simulink model "soc_WLAN_fpga"  (R2024b)
settings: Solver=FixedStepDiscrete  StartTime=0.0  StopTime=stopTime  RelTol=1e-3
PreLoadFcn:
  | addpath(fullfile(matlabroot,'toolbox','whdl','whdlexamples','whdlexamples'));
InitFcn:
  | addpath(fullfile(matlabroot,'toolbox','whdl','whdlexamples','whdlexamples'));
model workspace (MAT data in the model file):
  socvcb : containers.Map (value not decoded)
undefined symbols (not defined in the file): Add, bitRatePerOfdmSym, chanBW, coe, cpLen, dataUpsampleFactor, DelayValMaxNsdMinusLastPilotSc, DescramblerInitialSeed, designMultirateFIR, fftLen, filterLatency, filterUpsampleFactor, Fs, Hd, HT_MFMCS0, HT_MFMCS1, HT_MFMCS2, HT_MFMCS3, HT_MFMCS4, HT_MFMCS5, HT_MFMCS6, HT_MFMCS7, HTUnUsedScInd, inputSamplingRate, interp_coeff, maxPilotRefCounterVale, maxPilotsRef, maxPilotsRefNonHT, Ncol_HT, Ncol_NonHT, noDataSubCarriers, Non_HTMCS0, Non_HTMCS1, Non_HTMCS2, Non_HTMCS3, Non_HTMCS4, Non_HTMCS5, Non_HTMCS6, Non_HTMCS7, Nrow_HT, Nrow_NonHT, numDSC_HT, numDSC_HT_vhtSigB, numDSC_NonHT, numDscHT, numDscNonHT, numOfBitsPerOFDMSym, numOfDataBitsPerOFDMSym, numPilots, numScHT, numSCS_HT, numSCS_NonHT, pnSeq, QAM, rxDownsampleFactor, secondPIdx_HT, secondPIdx_NonHT, Shift, VHTMCS0, VHTMCS1 ... (+7)
libraries: hdlsllib x267, simulink x210, dspsigops x22, whdlutilities x10, whdlmod x9, dsphdlfiltering2 x5, dsphdlmathfun2 x4, whdledac x3, hwlogicconnlib x2, commhdlcrc x2, dsphdlsigops2 x2
(part 8 of 14)

== system soc_WLAN_fpga/WLAN/WLAN HDL/WLAN_Tx_Rx/WLAN_Rx/WLANHDLReceiver/FrameFormatDetectionAndSignalRecovery/SignalBitRecovery/Deinterleaver Block/Write Logic ==
  start : Inport
  valid : Inport  Port=2
  end : Inport  Port=3
  Generate Write Address : Subsystem
  Handle Input Control Signals : Subsystem
  wrAddr : Outport
  wrValid : Outport  Port=2
  count : Outport  Port=3
  endOut : Outport  Port=4
  endReady : Outport  Port=5
  wires:
  Handle Input Control Signals/4(endReady) -> endReady/1
  end/1 -> Handle Input Control Signals/3(end)
  valid/1 -> Handle Input Control Signals/2(valid)
  Generate Write Address/1(wrAddr) -> wrAddr/1
  Handle Input Control Signals/2(countEnb) -> Generate Write Address/2(enb), wrValid/1
  start/1 -> Handle Input Control Signals/1(start)
  Handle Input Control Signals/3(endOut) -> Generate Write Address/3(end), endOut/1
  Handle Input Control Signals/1(reset) -> Generate Write Address/1(rst)
  Generate Write Address/2(count) -> count/1

== system soc_WLAN_fpga/WLAN/WLAN HDL/WLAN_Tx_Rx/WLAN_Rx/WLANHDLReceiver/HT_VHTCPEEstAndCorrection/CPECorrector/Reciprocal/Function Impl ==
  switch : Inport
  LUTAddr : Inport  Port=2
  Delay{6..8,10,15..16} (6 alike) : Delay
  Delay9 : Delay  DelayLength=1
  LUT1 : LookupNDDirect  NumberOfTableDimensions=1  Table=LUT(:,1)  DiagnosticForOutOfRangeInput=Error
  LUT2 : LookupNDDirect  NumberOfTableDimensions=1  Table=LUT(:,2)  DiagnosticForOutOfRangeInput=Error
  Multiport Switch : MultiPortSwitch  DataPortOrder=Zero-based contiguous  Inputs=2  zeroidx=on  SaturateOnIntegerOverflow=off  InputSameDT=off
  functionValues : Outport
  wires:
  LUTAddr/1 -> Delay7/1, Delay6/1
  Delay15/1 -> Multiport Switch/2
  Delay16/1 -> Multiport Switch/3
  Delay10/1 -> Multiport Switch/1
  Delay9/1 -> functionValues/1
  LUT2/1 -> Delay15/1
  LUT1/1 -> Delay16/1
  switch/1 -> Delay8/1
  Delay8/1 -> Delay10/1
  Delay7/1 -> LUT2/1
  Delay6/1 -> LUT1/1
  Multiport Switch/1 -> Delay9/1

== system soc_WLAN_fpga/WLAN/WLAN HDL/WLAN_Tx_Rx/WLAN_Rx/WLANHDLReceiver/NonHTCPEEstAndCorrection/CPECorrector/Reciprocal/Function Impl ==
  switch : Inport
  LUTAddr : Inport  Port=2
  Delay{6..8,10,15..16} (6 alike) : Delay
  Delay9 : Delay  DelayLength=1
  LUT1 : LookupNDDirect  NumberOfTableDimensions=1  Table=LUT(:,1)  DiagnosticForOutOfRangeInput=Error
  LUT2 : LookupNDDirect  NumberOfTableDimensions=1  Table=LUT(:,2)  DiagnosticForOutOfRangeInput=Error
  Multiport Switch : MultiPortSwitch  DataPortOrder=Zero-based contiguous  Inputs=2  zeroidx=on  SaturateOnIntegerOverflow=off  InputSameDT=off
  functionValues : Outport
  wires:
  LUTAddr/1 -> Delay7/1, Delay6/1
  Delay15/1 -> Multiport Switch/2
  Delay16/1 -> Multiport Switch/3
  Delay10/1 -> Multiport Switch/1
  Delay9/1 -> functionValues/1
  LUT2/1 -> Delay15/1
  LUT1/1 -> Delay16/1
  switch/1 -> Delay8/1
  Delay8/1 -> Delay10/1
  Delay7/1 -> LUT2/1
  Delay6/1 -> LUT1/1
  Multiport Switch/1 -> Delay9/1

== system soc_WLAN_fpga/WLAN/WLAN HDL/WLAN_Tx_Rx/WLAN_Rx/WLANHDLReceiver/WLANTimeAndFrequencySynchronization/Coarse CFO Estimation and Correction/Coarse CFO Estimation/averager ==
  corrIn : Inport
  load : Inport  Port=2
  rst : Inport  Port=3
  Compare To Constant : simulink/Logic and Bit Operations/Compare To Constant  relop===  const=wlanConfig.lstfLen*10-1  OutDataTypeStr=boolean
  Compare To Constant1 : simulink/Logic and Bit Operations/Compare To Constant  relop=>=  const=round(wlanConfig.lstfLen*0.75)  OutDataTypeStr=boolean
  Compare To Constant2 : simulink/Logic and Bit Operations/Compare To Constant  relop=<=  const=round(wlanConfig.lstfLen*0.75)+8*wlanConfig.lstfLen-1  OutDataTypeStr=boolean
  Compare To Constant3 : simulink/Logic and Bit Operations/Compare To Constant  relop===  const=round(wlanConfig.lstfLen*0.75)+8*wlanConfig.lstfLen-1  OutDataTypeStr=boolean
  Compare To Zero : simulink/Logic and Bit Operations/Compare To Zero  relop=>  OutDataTypeStr=boolean
  Constant : Constant  OutDataTypeStr=uint16  SampleTime=-1
  Constant1 : Constant  Value=complex(0,0)  OutDataTypeStr=Inherit: Inherit via back propagation  SampleTime=-1
  Delay : Delay  DelayLength=1
  HDL Counter : hdlsllib/Sources/HDL Counter  CountType=Count limited  CountInit=0  CountStep=1  CountMax=10*wlanConfig.lstfLen-1  CountFromType=Initial value  CountFrom=0  CountResetPort=on  CountLoadPort=on  CountEnbPort=on  CountDirPort=off  CountHitOutputPort=off  CountDataType=Unsigned  CountWordLen=16  CountFracLen=0  CountSampTime=1
  Logical Operator : Logic  AllPortsSameDT=off  OutDataTypeStr=boolean
  Logical Operator1 : Logic  Operator=OR  AllPortsSameDT=off  OutDataTypeStr=boolean
  Sum : Sum
  Switch : Switch  Criteria=u2 ~= 0  Threshold=1  SaturateOnIntegerOverflow=off  InputSameDT=off
  avgCorr : Outport
  validOut : Outport  Port=2
  wires:
  HDL Counter/1 -> Compare To Constant2/1, Compare To Constant1/1, Compare To Zero/1, Compare To Constant/1, Compare To Constant3/1
  Compare To Constant2/1 -> Logical Operator/1
  Constant/1 -> HDL Counter/3
  Sum/1 -> avgCorr/1, Switch/1
  Constant1/1 -> Switch/3
  corrIn/1 -> Sum/2
  Compare To Zero/1 -> HDL Counter/4
  Logical Operator1/1 -> HDL Counter/1
  Compare To Constant1/1 -> Logical Operator/2
  Logical Operator/1 -> Switch/2
  Compare To Constant/1 -> Logical Operator1/1
  Delay/1 -> Sum/1
  Switch/1 -> Delay/1
  rst/1 -> Logical Operator1/2
  Compare To Constant3/1 -> validOut/1
  load/1 -> HDL Counter/2

== system soc_WLAN_fpga/WLAN/WLAN HDL/WLAN_Tx_Rx/WLAN_Rx/WLANHDLReceiver/WLANTimeAndFrequencySynchronization/Coarse CFO Estimation and Correction/Coarse CFO Estimation/correlator ==
  dataIn : Inport
  lstf_start : Inport  Port=2
  Data Type Conversion : DataTypeConversion  OutDataTypeStr=fixdt(1,31,19)  SaturateOnIntegerOverflow=off  RndMeth=Floor
  Delay1 : Delay  InitialCondition=0  UseCircularBuffer=on
  Delay2 : Delay  DelayLength=wlanConfig.lstfLen  InitialCondition=0
  Delay3 : Delay  InitialCondition=0  UseCircularBuffer=on
  Delay4 : Delay  DelayLength=wlanConfig.lstfLen  InitialCondition=0
  Delay5 : Delay  InitialCondition=0  UseCircularBuffer=on
  Product : Product  RndMeth=Round
  complexConj : Math  Operator=conj  SignedPower=on  SaturateOnIntegerOverflow=off
  corrOut : Outport
  load : Outport  Port=2
  wires:
  dataIn/1 -> Delay2/1, Delay1/1
  Delay1/1 -> Product/1
  Product/1 -> Data Type Conversion/1
  Delay2/1 -> complexConj/1
  Delay3/1 -> Product/2
  complexConj/1 -> Delay3/1
  Data Type Conversion/1 -> corrOut/1
  lstf_start/1 -> Delay4/1
  Delay4/1 -> Delay5/1
  Delay5/1 -> load/1

== system soc_WLAN_fpga/WLAN/WLAN HDL/WLAN_Tx_Rx/WLAN_Rx/WLANHDLReceiver/WLANTimeAndFrequencySynchronization/Coarse Time Sync/correlator/MagnitudeSquared ==
  dataIn : Inport
  validIn : Inport  Port=2
  Add : Sum  OutDataTypeStr=Inherit: Same as accumulator
  Complex to Real-Imag : ComplexToRealImag
  Data Type Conversion : DataTypeConversion  OutDataTypeStr=fixdt(1,32,25)  SaturateOnIntegerOverflow=off  RndMeth=Floor
  Delay{,1..3} (4 alike) : Delay
  Delay4 : Delay  DelayLength=1
  Delay5 : Delay  DelayLength=1
  Delay6 : Delay  DelayLength=3
  Product1 : Product  OutDataTypeStr=fixdt(1,32,28)
  Product4 : Product  OutDataTypeStr=fixdt(1,32,28)
  dataOut : Outport  VectorParamsAs1DForOutWhenUnconnected=off
  validOut : Outport  Port=2  VectorParamsAs1DForOutWhenUnconnected=off
  wires:
  Complex to Real-Imag/2 -> Delay3/1, Delay2/1
  dataIn/1 -> Data Type Conversion/1
  validIn/1 -> Delay6/1
  Complex to Real-Imag/1 -> Delay1/1, Delay/1
  Product4/1 -> Delay4/1
  Product1/1 -> Delay5/1
  Add/1 -> dataOut/1
  Delay/1 -> Product4/2
  Delay1/1 -> Product4/1
  Delay2/1 -> Product1/1
  Delay3/1 -> Product1/2
  Delay4/1 -> Add/1
  Delay5/1 -> Add/2
  Delay6/1 -> validOut/1
  Data Type Conversion/1 -> Complex to Real-Imag/1

== system soc_WLAN_fpga/WLAN/WLAN HDL/WLAN_Tx_Rx/WLAN_Rx/WLANHDLReceiver/WLANTimeAndFrequencySynchronization/Coarse Time Sync/correlator/MovingSum ==
  dataIn : Inport
  validIn : Inport  Port=2
  reset : Inport  Port=3
  Add : Sum  Inputs=|+-  OutDataTypeStr=Inherit: Same as accumulator
  Add1 : Sum  OutDataTypeStr=Inherit: Same as first input
  Delay{3..6,12} (5 alike) : Delay  DelayLength=1  InitialCondition=0
  Shift Arithmetic : ArithShift  BitShiftNumber=1  BitShiftDirection=Right
  "Synchronous Enabled 16 Sample Delay " : Subsystem
  Synchronous Enabled Unit Delay : hdlsllib/Discrete/Unit Delay Enabled Synchronous  InitialCondition=0.0  SampleTime=-1
  dataOut : Outport  VectorParamsAs1DForOutWhenUnconnected=off
  validOut : Outport  Port=2  VectorParamsAs1DForOutWhenUnconnected=off
  wires:
  "Synchronous Enabled 16 Sample Delay "/1(dataOut) -> Add/2
  Synchronous Enabled Unit Delay/1 -> Add1/1, Delay5/1
  dataIn/1 -> "Synchronous Enabled 16 Sample Delay "/1(dataIn), Add/1
  Delay6/1 -> validOut/1
  Delay5/1 -> dataOut/1
  Delay4/1 -> Delay6/1
  Delay3/1 -> Synchronous Enabled Unit Delay/2, Delay4/1
  validIn/1 -> Delay3/1, "Synchronous Enabled 16 Sample Delay "/2(en)
  Add/1 -> Shift Arithmetic/1
  Add1/1 -> Synchronous Enabled Unit Delay/1
  reset/1 -> "Synchronous Enabled 16 Sample Delay "/3(reset)
  Delay12/1 -> Add1/2
  Shift Arithmetic/1 -> Delay12/1

== system soc_WLAN_fpga/WLAN/WLAN HDL/WLAN_Tx_Rx/WLAN_Rx/WLANHDLReceiver/WLANTimeAndFrequencySynchronization/Coarse Time Sync/correlator/delayedCorrelation ==
  dataIn : Inport
  validIn : Inport  Port=2
  startIn : Inport  Port=3
  Conjugate : Math  Operator=conj  SignedPower=on  RndMeth=Zero
  DTadjust : MATLAB Function  TreatAsAtomicUnit=on
  Delay1 : Delay  DelayLength=wlanConfig.lstfLen
  Delay16 : Delay  DelayLength=wlanConfig.lstfLen
  Delay4 : Delay
  Delay5 : Delay
  Delay6 : Delay  DelayLength=1
  Delay7 : Delay  DelayLength=3
  Delay8 : Delay  DelayLength=3
  Product : Product
  corrOut : Outport
  corrValid : Outport  Port=2
  startOut : Outport  Port=3
  wires:
  dataIn/1 -> Delay4/1, Delay16/1
  Delay16/1 -> Conjugate/1
  Delay4/1 -> Product/1
  Conjugate/1 -> Delay5/1
  Delay5/1 -> Product/2
  startIn/1 -> Delay8/1
  Delay1/1 -> Delay7/1
  Product/1 -> Delay6/1
  validIn/1 -> Delay1/1
  Delay8/1 -> startOut/1
  Delay7/1 -> corrValid/1
  Delay6/1 -> DTadjust/1(in)
  DTadjust/1(out) -> corrOut/1

== system soc_WLAN_fpga/WLAN/WLAN HDL/WLAN_Tx_Rx/WLAN_Rx/WLANHDLReceiver/WLANTimeAndFrequencySynchronization/Coarse Time Sync/energyCalculator/magnitudeSquared ==
  dataIn : Inport
  validIn : Inport  Port=2
  Add : Sum
  Delay : Delay  DelayLength=wlanConfig.lstfLen
  Delay1 : Delay  DelayLength=wlanConfig.lstfLen
  Delay2 : Delay  DelayLength=wlanConfig.lstfLen-1
  Delay3 : Delay  DelayLength=1
  Delay4 : Delay  DelayLength=1
  MagnitudeSquared : Subsystem
  MagnitudeSquared1 : Subsystem
  MovingSum : Subsystem  InitFcn=Simulink.suppressDiagnostic(gcb, 'SimulinkFixedPoint:util:Overflowoccurred');
  Shift Arithmetic : ArithShift  BitShiftNumber=1  BitShiftDirection=Right
  Shift Arithmetic1 : ArithShift  BitShiftNumber=log2(wlanConfig.lstfLen)  BitShiftDirection=Right
  Shift Arithmetic2 : ArithShift  BitShiftNumber=1  BitShiftDirection=Right
  energy : Outport
  push : Outport  Port=2
  wires:
  validIn/1 -> MagnitudeSquared/2(validIn)
  dataIn/1 -> MagnitudeSquared/1(dataIn)
  MagnitudeSquared/1(dataOut) -> Delay3/1
  Delay/1 -> Add/2
  Add/1 -> Shift Arithmetic/1
  Shift Arithmetic/1 -> MovingSum/1(dataIn)
  MovingSum/1(dataOut) -> Shift Arithmetic1/1
  Shift Arithmetic1/1 -> MagnitudeSquared1/1(dataIn)
  Delay2/1 -> MagnitudeSquared1/2(validIn)
  MagnitudeSquared1/1(dataOut) -> Shift Arithmetic2/1
  MagnitudeSquared1/2(validOut) -> push/1
  Shift Arithmetic2/1 -> energy/1
  Delay1/1 -> MovingSum/2(validIn)
  Delay3/1 -> Delay/1, Add/1
  Delay4/1 -> Delay1/1
  MagnitudeSquared/2(validOut) -> Delay4/1
  MovingSum/2(validOut) -> Delay2/1

== system soc_WLAN_fpga/WLAN/WLAN HDL/WLAN_Tx_Rx/WLAN_Rx/WLANHDLReceiver/WLANTimeAndFrequencySynchronization/Coarse Time Sync/peakDetection/considerFirstPeak ==
  peakIn : Inport
  Compare To Constant : simulink/Logic and Bit Operations/Compare To Constant  relop===  const=wlanConfig.lstfLen*10-1  OutDataTypeStr=boolean
  Compare To Constant1 : simulink/Logic and Bit Operations/Compare To Constant  relop===  const=0  OutDataTypeStr=boolean
  Delay10 : Delay  DelayLength=1
  Delay7 : Delay  DelayLength=1
  Delay9 : Delay  DelayLength=1
  HDL Counter1 : hdlsllib/Sources/HDL Counter  CountType=Count limited  CountInit=0  CountStep=1  CountMax=wlanConfig.lstfLen*10-1  CountFromType=Initial value  CountFrom=0  CountResetPort=on  CountLoadPort=off  CountEnbPort=on  CountDirPort=off  CountHitOutputPort=off  CountDataType=Unsigned  CountWordLen=16  CountFracLen=0  CountSampTime=1
  Logical Operator1 : Logic  AllPortsSameDT=off  OutDataTypeStr=boolean
  Logical Operator2 : Logic  Operator=OR  AllPortsSameDT=off  OutDataTypeStr=boolean
  Logical Operator6 : Logic  Operator=OR  AllPortsSameDT=off  OutDataTypeStr=boolean
  Logical Operator7 : Logic  AllPortsSameDT=off  OutDataTypeStr=boolean
  Switch : Switch  Criteria=u2 ~= 0  SaturateOnIntegerOverflow=off  InputSameDT=off
  peakOut : Outport
  validOut : Outport  Port=2
  wires:
  Logical Operator6/1 -> Delay10/1, Delay9/1
  HDL Counter1/1 -> Compare To Constant/1, Compare To Constant1/1
  Logical Operator2/1 -> Delay7/1, validOut/1
  Logical Operator1/1 -> Logical Operator7/2, Switch/3, Logical Operator6/1, Logical Operator2/1
  Delay10/1 -> Switch/2, Logical Operator7/1
  Compare To Constant/1 -> HDL Counter1/1
  peakIn/1 -> Logical Operator1/2, HDL Counter1/2
  Delay7/1 -> Logical Operator2/2
  Delay9/1 -> Logical Operator6/2
  Logical Operator7/1 -> Switch/1
  Compare To Constant1/1 -> Logical Operator1/1
  Switch/1 -> peakOut/1

== system soc_WLAN_fpga/WLAN/WLAN HDL/WLAN_Tx_Rx/WLAN_Rx/WLANHDLReceiver/WLANTimeAndFrequencySynchronization/Fine CFO Estimation and Correction/Fine CFO Estimation/averaging unit ==
  corrIn : Inport
  rst : Inport  Port=2
  load : Inport  Port=3
  Compare To Constant : simulink/Logic and Bit Operations/Compare To Constant  relop===  const=wlanConfig.lltfLen*2-1  OutDataTypeStr=boolean
  Compare To Constant1 : simulink/Logic and Bit Operations/Compare To Constant  relop=>=  const=round(wlanConfig.lstfLen*2*0.75)  OutDataTypeStr=boolean
  Compare To Constant2 : simulink/Logic and Bit Operations/Compare To Constant  relop=<=  const=round(wlanConfig.lstfLen*2*0.75)+wlanConfig.lstfLen*4-1  OutDataTypeStr=boolean
  Compare To Constant3 : simulink/Logic and Bit Operations/Compare To Constant  relop===  const=round(wlanConfig.lstfLen*2*0.75)+wlanConfig.lstfLen*4-1  OutDataTypeStr=boolean
  Compare To Zero : simulink/Logic and Bit Operations/Compare To Zero  relop=>  OutDataTypeStr=boolean
  Constant : Constant  OutDataTypeStr=uint16  SampleTime=-1
  Constant1 : Constant  Value=complex(0,0)  OutDataTypeStr=Inherit: Inherit via back propagation  SampleTime=-1
  Delay : Delay  DelayLength=1
  HDL Counter : hdlsllib/Sources/HDL Counter  CountType=Count limited  CountInit=0  CountStep=1  CountMax=2*wlanConfig.lltfLen-1  CountFromType=Initial value  CountFrom=0  CountResetPort=on  CountLoadPort=on  CountEnbPort=on  CountDirPort=off  CountHitOutputPort=off  CountDataType=Unsigned  CountWordLen=16  CountFracLen=0  CountSampTime=1
  Logical Operator : Logic  AllPortsSameDT=off  OutDataTypeStr=boolean
  Logical Operator1 : Logic  Operator=OR  AllPortsSameDT=off  OutDataTypeStr=boolean
  Sum : Sum
  Switch : Switch  Criteria=u2 ~= 0  Threshold=1  SaturateOnIntegerOverflow=off  InputSameDT=off
  avgCorr : Outport
  validOut : Outport  Port=2
  wires:
  Constant/1 -> HDL Counter/3
  HDL Counter/1 -> Compare To Constant1/1, Compare To Zero/1, Compare To Constant2/1, Compare To Constant/1, Compare To Constant3/1
  Sum/1 -> avgCorr/1, Switch/1
  Compare To Zero/1 -> HDL Counter/4
  Compare To Constant1/1 -> Logical Operator/2
  rst/1 -> Logical Operator1/2
  Compare To Constant2/1 -> Logical Operator/1
  Constant1/1 -> Switch/3
  Logical Operator/1 -> Switch/2
  corrIn/1 -> Sum/2
  Switch/1 -> Delay/1
  Delay/1 -> Sum/1
  Compare To Constant/1 -> Logical Operator1/1
  Logical Operator1/1 -> HDL Counter/1
  load/1 -> HDL Counter/2
  Compare To Constant3/1 -> validOut/1

== system soc_WLAN_fpga/WLAN/WLAN HDL/WLAN_Tx_Rx/WLAN_Rx/WLANHDLReceiver/WLANTimeAndFrequencySynchronization/Fine CFO Estimation and Correction/Fine CFO Estimation/correlator ==
  dataIn : Inport
  Data Type Conversion : DataTypeConversion  OutDataTypeStr=fixdt(1,31,19)  SaturateOnIntegerOverflow=off  RndMeth=Floor
  Data Type Conversion1 : DataTypeConversion  OutDataTypeStr=fixdt(1,16,12)  SaturateOnIntegerOverflow=off  RndMeth=Floor
  Delay1 : Delay  InitialCondition=0  UseCircularBuffer=on
  Delay2 : Delay  DelayLength=wlanConfig.lstfLen*4  InitialCondition=0
  Delay3 : Delay  InitialCondition=0  UseCircularBuffer=on
  Delay32 : Delay  DelayLength=1
  Product : Product  RndMeth=Round
  complexConj : Math  Operator=conj  SignedPower=on  SaturateOnIntegerOverflow=off
  corrOut : Outport
  wires:
  Data Type Conversion/1 -> corrOut/1
  Delay1/1 -> Product/1
  Delay2/1 -> complexConj/1
  complexConj/1 -> Delay3/1
  Delay32/1 -> Data Type Conversion/1
  Data Type Conversion1/1 -> Delay1/1, Delay2/1
  Delay3/1 -> Product/2
  Product/1 -> Delay32/1
  dataIn/1 -> Data Type Conversion1/1

== system soc_WLAN_fpga/WLAN/WLAN HDL/WLAN_Tx_Rx/WLAN_Rx/WLANHDLReceiver/WLANTimeAndFrequencySynchronization/Fine Time Sync/correlator/MagnitudeSquared ==
  dataIn : Inport
  validIn : Inport  Port=2
  Add : Sum  OutDataTypeStr=Inherit: Same as accumulator
  Complex to Real-Imag : ComplexToRealImag
  Data Type Conversion : DataTypeConversion  OutDataTypeStr=fixdt(1,16,8)  SaturateOnIntegerOverflow=off  RndMeth=Floor
  Data Type Conversion1 : DataTypeConversion  OutDataTypeStr=fixdt(1,32,15)  SaturateOnIntegerOverflow=off  RndMeth=Floor
  Delay{,1..3} (4 alike) : Delay
  Delay4 : Delay  DelayLength=1
  Delay5 : Delay  DelayLength=1
  Delay6 : Delay  DelayLength=3
  Product1 : Product
  Product4 : Product
  dataOut : Outport  VectorParamsAs1DForOutWhenUnconnected=off
  validOut : Outport  Port=2  VectorParamsAs1DForOutWhenUnconnected=off
  wires:
  Complex to Real-Imag/2 -> Delay3/1, Delay2/1
  validIn/1 -> Delay6/1
  Complex to Real-Imag/1 -> Delay1/1, Delay/1
  Product4/1 -> Delay4/1
  Product1/1 -> Delay5/1
  Delay4/1 -> Add/1
  Delay5/1 -> Add/2
  Delay6/1 -> validOut/1
  dataIn/1 -> Data Type Conversion/1
  Delay1/1 -> Product4/2
  Delay2/1 -> Product1/1
  Delay3/1 -> Product1/2
  Delay/1 -> Product4/1
  Data Type Conversion/1 -> Complex to Real-Imag/1
  Data Type Conversion1/1 -> dataOut/1
  Add/1 -> Data Type Conversion1/1

== system soc_WLAN_fpga/WLAN/WLAN HDL/WLAN_Tx_Rx/WLAN_Rx/WLANHDLReceiver/WLANTimeAndFrequencySynchronization/Fine Time Sync/correlator/corrFilter ==
  note: Upsample by 8 for 20MHz and 4 for 40MHz is used for 'Resource Sharing' in the Discrete FIR filter
  note: delayLen=filterUpsampleFactor-1
  note: Latency = (coeffLen/filterUpsampleFactor)+filterUpsampleFactor+9
  dataIn : Inport
  validIn : Inport  Port=2
  rst : Inport  Port=3
  C1 : dsphdlfiltering2/Discrete FIR Filter  NumeratorSource=Property  Numerator=conj(flipud(wlanConfig.lltf(1:wlanConfig.corrLen))).'  NumeratorPrototype=[ 0.5, 0.5 ]  FilterStructure=Partly serial systolic  SerializationOption=Minimum number of cycles between valid input samples  NumCycles=filterUpsampleFactor  NumberOfMultipliers=2  SimulateUsing=Code generation  roundingMode=Floor  overflowMode=off  CoefficientsDataTypeStr=fixdt(1,16,14)  ResetInputPort=on  HDLGlobalReset=off  CoeffMultiplier=Multiplier  UseMultForPow2Coeff=on
  Delay : Delay  DelayLength=filterUpsampleFactor-1
  Delay1 : Delay  DelayLength=filterUpsampleFactor-1
  Delay2 : Delay  DelayLength=filterUpsampleFactor-1
  Downsample : DownSample  N=filterUpsampleFactor  RateOptions=Allow multirate processing
  Downsample1 : DownSample  N=filterUpsampleFactor  RateOptions=Allow multirate processing
  Terminator : Terminator
  Upsample : dspsigops/Upsample  FactorSource=Dialog parameter  N=filterUpsampleFactor  Nmax=16  phase=0  RateOptions=Allow multirate processing  ic=0  mode=Unused parameter value
  Upsample1 : dspsigops/Upsample  FactorSource=Dialog parameter  N=filterUpsampleFactor  Nmax=16  phase=0  RateOptions=Allow multirate processing  ic=0  mode=Unused parameter value
  Upsample2 : dspsigops/Upsample  FactorSource=Dialog parameter  N=filterUpsampleFactor  Nmax=16  phase=0  RateOptions=Allow multirate processing  ic=0  mode=Unused parameter value
  dataOut : Outport
  validOut : Outport  Port=2
  wires:
  dataIn/1 -> Upsample/1
  validIn/1 -> Upsample1/1
  Upsample1/1 -> C1/2
  C1/2 -> Delay1/1
  C1/3 -> Delay2/1
  Delay/1 -> Downsample/1
  Delay1/1 -> Downsample1/1
  Delay2/1 -> Terminator/1
  Downsample/1 -> dataOut/1
  Downsample1/1 -> validOut/1
  Upsample/1 -> C1/1
  C1/1 -> Delay/1
  rst/1 -> Upsample2/1
  Upsample2/1 -> C1/3

== system soc_WLAN_fpga/WLAN/WLAN HDL/WLAN_Tx_Rx/WLAN_Rx/WLANHDLReceiver/WLANTimeAndFrequencySynchronization/Fine Time Sync/peakSearcher/maxPeakSearcher ==
  corrIn : Inport
  corrValid : Inport  Port=2
  startIn : Inport  Port=3
  validIn : Inport  Port=4
  dataIn : Inport  Port=5
  rstIn : Inport  Port=6
  Delay1 : Delay  DelayLength=wlanConfig.lltfLen-1
  Delay{2,27..32} (7 alike) : Delay  DelayLength=1
  Delay3 : Delay  DelayLength=wlanConfig.lltfLen-1
  Delay4 : Delay  DelayLength=2*wlanConfig.corrLen+1
  Delay6 : Delay  DelayLength=2*wlanConfig.corrLen+1
  Delay8 : Delay  DelayLength=2*wlanConfig.corrLen+1
  Delay9 : Delay  DelayLength=wlanConfig.lltfLen-1
  Logical Operator : Logic  Operator=OR  AllPortsSameDT=off  OutDataTypeStr=boolean
  extractLTFs : Subsystem
  maxPeakSearcher : MATLAB Function  TreatAsAtomicUnit=on
  maxPeakValue : Outport
  countRst : Outport  Port=2
  dataOut : Outport  Port=3
  validOut : Outport  Port=4
  wires:
  Delay9/1 -> Delay31/1, Delay30/1
  Logical Operator/1 -> Delay9/1, extractLTFs/2(rst)
  extractLTFs/1(valid) -> Delay28/1
  Delay27/1 -> maxPeakSearcher/1(dataIn)
  Delay31/1 -> Delay8/1
  Delay30/1 -> maxPeakSearcher/4(reset)
  Delay29/1 -> maxPeakSearcher/3(countValue)
  extractLTFs/2(count) -> Delay29/1
  Delay28/1 -> maxPeakSearcher/2(validIn)
  maxPeakSearcher/1(maxPeak) -> maxPeakValue/1
  corrValid/1 -> extractLTFs/1(enb)
  corrIn/1 -> Delay27/1
  Delay32/1 -> Delay6/1
  Delay3/1 -> Delay32/1
  validIn/1 -> Delay3/1
  Delay6/1 -> validOut/1
  Delay2/1 -> Delay4/1
  Delay1/1 -> Delay2/1
  dataIn/1 -> Delay1/1
  Delay4/1 -> dataOut/1
  Delay8/1 -> countRst/1
  rstIn/1 -> Logical Operator/1
  startIn/1 -> Logical Operator/2

== system soc_WLAN_fpga/WLAN/WLAN HDL/WLAN_Tx_Rx/WLAN_Rx/WLANHDLReceiver/WLANTimeAndFrequencySynchronization/Fine Time Sync/peakSearcher/peakDetector ==
  maxPeakVal : Inport
  counterRst : Inport  Port=2
  dataIn : Inport  Port=3
  validIn : Inport  Port=4
  Delay{7,10,12,17..18,20..21} (7 alike) : Delay  DelayLength=1
  HDL Counter2 : hdlsllib/Sources/HDL Counter  CountType=Count limited  CountInit=0  CountStep=1  CountMax=2^16-1  CountFromType=Initial value  CountFrom=0  CountResetPort=on  CountLoadPort=off  CountEnbPort=on  CountDirPort=off  CountHitOutputPort=off  CountDataType=Unsigned  CountWordLen=16  CountFracLen=0  CountSampTime=1
  Logical Operator2 : Logic  Operator=OR  AllPortsSameDT=off  OutDataTypeStr=boolean
  Logical Operator3 : Logic  AllPortsSameDT=off  OutDataTypeStr=boolean
  Logical Operator4 : Logic  AllPortsSameDT=off  OutDataTypeStr=boolean
  Logical Operator6 : Logic  Operator=OR  AllPortsSameDT=off  OutDataTypeStr=boolean
  Logical Operator7 : Logic  AllPortsSameDT=off  OutDataTypeStr=boolean
  Relational Operator : RelationalOperator  Operator===  OutDataTypeStr=boolean  RndMeth=Simplest  InputSameDT=off
  Switch : Switch  Criteria=u2 ~= 0  SaturateOnIntegerOverflow=off  InputSameDT=off
  "dataSelector " : MATLAB Function  TreatAsAtomicUnit=on
  lstfStart : Outport
  validOut : Outport  Port=2
  dataOut : Outport  Port=3
  wires:
  Relational Operator/1 -> Logical Operator4/1
  Logical Operator3/1 -> validOut/1, "dataSelector "/1(syncEn)
  Logical Operator6/1 -> Delay12/1, Delay10/1
  Logical Operator2/1 -> Delay7/1, Logical Operator3/1
  Delay21/1 -> "dataSelector "/3(validIn), Logical Operator3/2, Logical Operator4/2
  Delay10/1 -> Switch/2, Logical Operator7/1
  Delay7/1 -> Logical Operator2/2
  Delay17/1 -> Relational Operator/1
  Logical Operator4/1 -> Logical Operator2/1, Switch/3, Logical Operator7/2, Logical Operator6/1
  Delay20/1 -> "dataSelector "/2(dataIn)
  Delay12/1 -> Logical Operator6/2
  dataIn/1 -> Delay20/1
  "dataSelector "/1(dataOut) -> dataOut/1
  Delay18/1 -> Relational Operator/2
  HDL Counter2/1 -> Delay18/1
  maxPeakVal/1 -> Delay17/1
  Switch/1 -> lstfStart/1
  counterRst/1 -> HDL Counter2/1
  validIn/1 -> HDL Counter2/2, Delay21/1
  Logical Operator7/1 -> Switch/1

== system soc_WLAN_fpga/WLAN/WLAN HDL/WLAN_Tx_Rx/WLAN_Rx/WLANHDLReceiver/DataRecovery/Decoder/vhtSigB/vhtSigBDecoding/vitInputLenCalc ==
  note: 1/(numSCs*modOrder*codeRate)
  note: numSCs*modOrder*codeRate
  note: numSCs*modOrder
  MCS : Inport
  psduLen : Inport  Port=2
  1-D Lookup Table : Lookup_n-D  NumberOfTableDimensions=1  BreakpointsForDimension1=[0:7]  IndexSearchMethod=Evenly spaced points  Table=numOfBitsPerOFDMSym  TableDataTypeStr=fixdt(0,16,0)  ExtrapMethod=Clip  UseLastTableValue=on  InternalRulePriority=Speed  OutDataTypeStr=fixdt(0,16,0)  RndMeth=Simplest
  1-D Lookup Table1 : Lookup_n-D  NumberOfTableDimensions=1  BreakpointsForDimension1=[0:7]  IndexSearchMethod=Evenly spaced points  Table=numOfDataBitsPerOFDMSym  TableDataTypeStr=fixdt(0,16,0)  ExtrapMethod=Clip  UseLastTableValue=on  InternalRulePriority=Speed  OutDataTypeStr=fixdt(0,16,0)  RndMeth=Simplest
  1-D Lookup Table2 : Lookup_n-D  NumberOfTableDimensions=1  BreakpointsForDimension1=[0:7]  IndexSearchMethod=Evenly spaced points  Table=bitRatePerOfdmSym  TableDataTypeStr=fixdt(0,20,20)  ExtrapMethod=Clip  UseLastTableValue=on  InternalRulePriority=Speed  OutDataTypeStr=fixdt(0,20,20)  RndMeth=Simplest
  Add : Sum
  Add1 : Sum  OutDataTypeStr=Inherit: Same as first input
  Add2 : Sum  Inputs=+-
  Constant : Constant  Value=fi(numDSC_HT,0,8,0)  SampleTime=-1
  Constant1 : Constant  Value=fi(22,0,5,0)  SampleTime=-1
  Constant2 : Constant  Value=fi(0.125,0,7,6)  SampleTime=-1
  Data Type Conversion : DataTypeConversion  OutDataTypeStr=uint16  RndMeth=Ceiling  SaturateOnIntegerOverflow=off
  Data Type Conversion : DataTypeConversion  OutDataTypeStr=fixdt(0,14,0)  SaturateOnIntegerOverflow=off  RndMeth=Floor
  Delay{,1..6} (7 alike) : Delay
  Delay{7..11} (5 alike) : Delay  DelayLength=1
  Delay12 : Delay  DelayLength=3
  Delay13 : Delay  DelayLength=3
  Product1 : Product  OutDataTypeStr=fixdt(0,17,0)  RndMeth=Ceiling
  Product2 : Product  RndMeth=Ceiling  OutDataTypeStr=Inherit: Same as first input
  Product3 : Product  RndMeth=Ceiling
  Product4 : Product  OutDataTypeStr=fixdt(1,32,20)  RndMeth=Ceiling
  Shift Arithmetic : ArithShift  BitShiftNumber=3  BitShiftDirection=Left
  updatedPsduLen : Outport
  decoderInpLen : Outport  Port=2
  wires:
  MCS/1 -> 1-D Lookup Table2/1, 1-D Lookup Table1/1, 1-D Lookup Table/1
  psduLen/1 -> Shift Arithmetic/1
  Shift Arithmetic/1 -> Add/1
  Constant1/1 -> Add/2, Delay11/1
  Constant/1 -> Add1/2
  Add/1 -> Delay/1
  Product4/1 -> Delay7/1
  Product1/1 -> Delay8/1
  Add1/1 -> Delay12/1  "inputLen"
  Add2/1 -> Delay5/1
  Product3/1 -> Delay10/1
  Data Type Conversion/1 -> Delay13/1
  Product2/1 -> Delay9/1
  1-D Lookup Table/1 -> Delay3/1
  1-D Lookup Table2/1 -> Delay1/1
  1-D Lookup Table1/1 -> Delay4/1
  Constant2/1 -> Delay6/1
  Delay/1 -> Product4/1
  Delay1/1 -> Product4/2
  Delay2/1 -> Product1/1, Product2/1
  Delay3/1 -> Product1/2
  Delay4/1 -> Product2/2
  Delay5/1 -> Product3/1
  Delay6/1 -> Product3/2
  Delay7/1 -> Data Type Conversion/1
  Delay8/1 -> Add1/1
  Delay10/1 -> Data Type Conversion/1
  Delay9/1 -> Add2/1
  Delay11/1 -> Add2/2
  Delay12/1 -> decoderInpLen/1
  Delay13/1 -> updatedPsduLen/1
  Data Type Conversion/1 -> Delay2/1  "numSymbols"

== system soc_WLAN_fpga/WLAN/WLAN HDL/WLAN_Tx_Rx/WLAN_Rx/WLANHDLReceiver/DataRecovery/Deinterleaver/DeInterleaver_HT/Stage 2 16QAM /Generate Ready ==
  advPop : Inport
  fifoCount : Inport  Port=2
  pop : Inport  Port=3
  endReady : Inport  Port=4
  Generate Ready2 : Subsystem
  Logical Operator1 : Logic  IconShape=distinctive  AllPortsSameDT=off  OutDataTypeStr=boolean
  Logical Operator2 : Logic  IconShape=distinctive  AllPortsSameDT=off  OutDataTypeStr=boolean
  Logical Operator3 : Logic  Operator=NOT  IconShape=distinctive  AllPortsSameDT=off  OutDataTypeStr=boolean
  MATLAB Function1 : MATLAB Function  TreatAsAtomicUnit=on  mask{nClocks=4}
      mask prompts: nClocks "Number of clocks to hold:"
  ready : Outport
  wires:
  pop/1 -> Generate Ready2/2(pop)
  Logical Operator3/1 -> Logical Operator2/2
  endReady/1 -> Logical Operator1/2
  MATLAB Function1/1(out) -> Logical Operator3/1
  fifoCount/1 -> Generate Ready2/1(fifoCount)
  Logical Operator1/1 -> MATLAB Function1/1(trigger)
  advPop/1 -> Logical Operator1/1
  Logical Operator2/1 -> ready/1
  Generate Ready2/1(ready2) -> Logical Operator2/1

== system soc_WLAN_fpga/WLAN/WLAN HDL/WLAN_Tx_Rx/WLAN_Rx/WLANHDLReceiver/DataRecovery/Deinterleaver/DeInterleaver_HT/Stage 2 16QAM /Read Logic ==
  fifoData : Inport
  fifoCount : Inport  Port=2
  Add1 : Sum  OutDataTypeStr=Inherit: Inherit via back propagation
  Delay1 : Delay  DelayLength=5
  Delay2 : Delay  DelayLength=5
  Delay3 : Delay  DelayLength=1
  Delay4 : Delay  DelayLength=5
  Delay7 : Delay  DelayLength=1
  Generate Base Read Address : Subsystem
  Generate Output Control Signals : Subsystem
  Generate Read Address : Subsystem  Variant=on
  MATLAB Function : MATLAB Function  TreatAsAtomicUnit=on  mask{nClocks=maxBlkSize}
      mask prompts: nClocks "Number of clocks to hold:"
  Relational Operator1 : RelationalOperator  Operator=<  OutDataTypeStr=boolean  InputSameDT=off
  Unit Delay Enabled Synchronous1 : hdlsllib/Discrete/Unit Delay Enabled Synchronous  InitialCondition=maxBlkSize -1  SampleTime=-1
  rdAddr : Outport
  start : Outport  Port=2
  end : Outport  Port=3
  valid : Outport  Port=4
  pop : Outport  Port=5
  advPop : Outport  Port=6
  wires:
  Generate Output Control Signals/5(advPop) -> advPop/1
  Generate Output Control Signals/4(pop) -> pop/1
  Delay1/1 -> Add1/2
  Generate Read Address/1(blockDataCount) -> Generate Output Control Signals/3(blockCount)
  Delay2/1 -> Generate Output Control Signals/2(blockValid)
  Delay4/1 -> Generate Output Control Signals/1(blockLen)
  Delay7/1 -> rdAddr/1
  Generate Output Control Signals/3(valid) -> valid/1
  Generate Output Control Signals/2(end) -> end/1
  Generate Output Control Signals/1(start) -> start/1
  Generate Read Address/2(currentAddr) -> Add1/1
  Generate Base Read Address/1(baseAddr) -> Delay1/1
  fifoData/1 -> Unit Delay Enabled Synchronous1/1
  Add1/1 -> Delay7/1
  Delay3/1 -> Relational Operator1/2
  MATLAB Function/1(out) -> Generate Read Address/2(enable), Delay2/1
  Unit Delay Enabled Synchronous1/1 -> Generate Read Address/1(blockLen), Delay4/1  "blockLen"
  Relational Operator1/1 -> Generate Read Address/3(reset), Generate Base Read Address/1(readStart), Unit Delay Enabled Synchronous1/2, MATLAB Function/1(trigger)  "readStart"
  fifoCount/1 -> Relational Operator1/1, Delay3/1

== system soc_WLAN_fpga/WLAN/WLAN HDL/WLAN_Tx_Rx/WLAN_Rx/WLANHDLReceiver/DataRecovery/Deinterleaver/DeInterleaver_HT/Stage 2 16QAM /Write Logic ==
  start : Inport
  valid : Inport  Port=2
  end : Inport  Port=3
  Generate Write Address : Subsystem
  Handle Input Control Signals : Subsystem
  wrAddr : Outport
  wrValid : Outport  Port=2
  count : Outport  Port=3
  endOut : Outport  Port=4
  endReady : Outport  Port=5
  wires:
  Handle Input Control Signals/4(endReady) -> endReady/1
  end/1 -> Handle Input Control Signals/3(end)
  valid/1 -> Handle Input Control Signals/2(valid)
  Generate Write Address/1(wrAddr) -> wrAddr/1
  Handle Input Control Signals/2(countEnb) -> Generate Write Address/2(enb), wrValid/1
  start/1 -> Handle Input Control Signals/1(start)
  Handle Input Control Signals/3(endOut) -> Generate Write Address/3(end), endOut/1
  Handle Input Control Signals/1(reset) -> Generate Write Address/1(rst)
  Generate Write Address/2(count) -> count/1

== system soc_WLAN_fpga/WLAN/WLAN HDL/WLAN_Tx_Rx/WLAN_Rx/WLANHDLReceiver/DataRecovery/Deinterleaver/DeInterleaver_HT/Stage 2 64QAM/Generate Ready ==
  advPop : Inport
  fifoCount : Inport  Port=2
  pop : Inport  Port=3
  endReady : Inport  Port=4
  Generate Ready2 : Subsystem
  Logical Operator1 : Logic  IconShape=distinctive  AllPortsSameDT=off  OutDataTypeStr=boolean
  Logical Operator2 : Logic  IconShape=distinctive  AllPortsSameDT=off  OutDataTypeStr=boolean
  Logical Operator3 : Logic  Operator=NOT  IconShape=distinctive  AllPortsSameDT=off  OutDataTypeStr=boolean
  MATLAB Function1 : MATLAB Function  TreatAsAtomicUnit=on  mask{nClocks=4}
      mask prompts: nClocks "Number of clocks to hold:"
  ready : Outport
  wires:
  pop/1 -> Generate Ready2/2(pop)
  Logical Operator3/1 -> Logical Operator2/2
  endReady/1 -> Logical Operator1/2
  MATLAB Function1/1(out) -> Logical Operator3/1
  fifoCount/1 -> Generate Ready2/1(fifoCount)
  Logical Operator1/1 -> MATLAB Function1/1(trigger)
  advPop/1 -> Logical Operator1/1
  Logical Operator2/1 -> ready/1
  Generate Ready2/1(ready2) -> Logical Operator2/1

== system soc_WLAN_fpga/WLAN/WLAN HDL/WLAN_Tx_Rx/WLAN_Rx/WLANHDLReceiver/DataRecovery/Deinterleaver/DeInterleaver_HT/Stage 2 64QAM/Read Logic ==
  fifoData : Inport
  fifoCount : Inport  Port=2
  Add1 : Sum  OutDataTypeStr=Inherit: Inherit via back propagation
  Delay1 : Delay  DelayLength=5
  Delay2 : Delay  DelayLength=5
  Delay3 : Delay  DelayLength=1
  Delay4 : Delay  DelayLength=5
  Delay7 : Delay  DelayLength=1
  Generate Base Read Address : Subsystem
  Generate Output Control Signals : Subsystem
  Generate Read Address : Subsystem  Variant=on
  MATLAB Function : MATLAB Function  TreatAsAtomicUnit=on  mask{nClocks=maxBlkSize}
      mask prompts: nClocks "Number of clocks to hold:"
  Relational Operator1 : RelationalOperator  Operator=<  OutDataTypeStr=boolean  InputSameDT=off
  Unit Delay Enabled Synchronous1 : hdlsllib/Discrete/Unit Delay Enabled Synchronous  InitialCondition=maxBlkSize -1  SampleTime=-1
  rdAddr : Outport
  start : Outport  Port=2
  end : Outport  Port=3
  valid : Outport  Port=4
  pop : Outport  Port=5
  advPop : Outport  Port=6
  wires:
  Generate Output Control Signals/5(advPop) -> advPop/1
  Generate Output Control Signals/4(pop) -> pop/1
  Delay1/1 -> Add1/2
  Generate Read Address/1(blockDataCount) -> Generate Output Control Signals/3(blockCount)
  Delay2/1 -> Generate Output Control Signals/2(blockValid)
  Delay4/1 -> Generate Output Control Signals/1(blockLen)
  Delay7/1 -> rdAddr/1
  Generate Output Control Signals/3(valid) -> valid/1
  Generate Output Control Signals/2(end) -> end/1
  Generate Output Control Signals/1(start) -> start/1
  Generate Read Address/2(currentAddr) -> Add1/1
  Generate Base Read Address/1(baseAddr) -> Delay1/1
  fifoData/1 -> Unit Delay Enabled Synchronous1/1
  Add1/1 -> Delay7/1
  Delay3/1 -> Relational Operator1/2
  MATLAB Function/1(out) -> Generate Read Address/2(enable), Delay2/1
  Unit Delay Enabled Synchronous1/1 -> Generate Read Address/1(blockLen), Delay4/1  "blockLen"
  Relational Operator1/1 -> Generate Read Address/3(reset), Generate Base Read Address/1(readStart), Unit Delay Enabled Synchronous1/2, MATLAB Function/1(trigger)  "readStart"
  fifoCount/1 -> Relational Operator1/1, Delay3/1

== system soc_WLAN_fpga/WLAN/WLAN HDL/WLAN_Tx_Rx/WLAN_Rx/WLANHDLReceiver/DataRecovery/Deinterleaver/DeInterleaver_HT/Stage 2 64QAM/Write Logic ==
  start : Inport
  valid : Inport  Port=2
  end : Inport  Port=3
  Generate Write Address : Subsystem
  Handle Input Control Signals : Subsystem
  wrAddr : Outport
  wrValid : Outport  Port=2
  count : Outport  Port=3
  endOut : Outport  Port=4
  endReady : Outport  Port=5
  wires:
  Handle Input Control Signals/4(endReady) -> endReady/1
  end/1 -> Handle Input Control Signals/3(end)
  valid/1 -> Handle Input Control Signals/2(valid)
  Generate Write Address/1(wrAddr) -> wrAddr/1
  Handle Input Control Signals/2(countEnb) -> Generate Write Address/2(enb), wrValid/1
  start/1 -> Handle Input Control Signals/1(start)
  Handle Input Control Signals/3(endOut) -> Generate Write Address/3(end), endOut/1
  Handle Input Control Signals/1(reset) -> Generate Write Address/1(rst)
  Generate Write Address/2(count) -> count/1

== system soc_WLAN_fpga/WLAN/WLAN HDL/WLAN_Tx_Rx/WLAN_Rx/WLANHDLReceiver/DataRecovery/Deinterleaver/DeInterleaver_HT/Stage 2 BPSK/Generate Ready ==
  advPop : Inport
  fifoCount : Inport  Port=2
  pop : Inport  Port=3
  endReady : Inport  Port=4
  Generate Ready2 : Subsystem
  Logical Operator1 : Logic  IconShape=distinctive  AllPortsSameDT=off  OutDataTypeStr=boolean
  Logical Operator2 : Logic  IconShape=distinctive  AllPortsSameDT=off  OutDataTypeStr=boolean
  Logical Operator3 : Logic  Operator=NOT  IconShape=distinctive  AllPortsSameDT=off  OutDataTypeStr=boolean
  MATLAB Function1 : MATLAB Function  TreatAsAtomicUnit=on  mask{nClocks=4}
      mask prompts: nClocks "Number of clocks to hold:"
  ready : Outport
  wires:
  pop/1 -> Generate Ready2/2(pop)
  Logical Operator3/1 -> Logical Operator2/2
  endReady/1 -> Logical Operator1/2
  MATLAB Function1/1(out) -> Logical Operator3/1
  fifoCount/1 -> Generate Ready2/1(fifoCount)
  Logical Operator1/1 -> MATLAB Function1/1(trigger)
  advPop/1 -> Logical Operator1/1
  Logical Operator2/1 -> ready/1
  Generate Ready2/1(ready2) -> Logical Operator2/1

== system soc_WLAN_fpga/WLAN/WLAN HDL/WLAN_Tx_Rx/WLAN_Rx/WLANHDLReceiver/DataRecovery/Deinterleaver/DeInterleaver_HT/Stage 2 BPSK/Read Logic ==
  fifoData : Inport
  fifoCount : Inport  Port=2
  Add1 : Sum  OutDataTypeStr=Inherit: Inherit via back propagation
  Delay1 : Delay  DelayLength=5
  Delay2 : Delay  DelayLength=5
  Delay3 : Delay  DelayLength=1
  Delay4 : Delay  DelayLength=5
  Delay7 : Delay  DelayLength=1
  Generate Base Read Address : Subsystem
  Generate Output Control Signals : Subsystem
  Generate Read Address : Subsystem  Variant=on
  MATLAB Function : MATLAB Function  TreatAsAtomicUnit=on  mask{nClocks=maxBlkSize}
      mask prompts: nClocks "Number of clocks to hold:"
  Relational Operator1 : RelationalOperator  Operator=<  OutDataTypeStr=boolean  InputSameDT=off
  Unit Delay Enabled Synchronous1 : hdlsllib/Discrete/Unit Delay Enabled Synchronous  InitialCondition=maxBlkSize -1  SampleTime=-1
  rdAddr : Outport
  start : Outport  Port=2
  end : Outport  Port=3
  valid : Outport  Port=4
  pop : Outport  Port=5
  advPop : Outport  Port=6
  wires:
  Generate Output Control Signals/5(advPop) -> advPop/1
  Generate Output Control Signals/4(pop) -> pop/1
  Delay1/1 -> Add1/2
  Generate Read Address/1(blockDataCount) -> Generate Output Control Signals/3(blockCount)
  Delay2/1 -> Generate Output Control Signals/2(blockValid)
  Delay4/1 -> Generate Output Control Signals/1(blockLen)
  Delay7/1 -> rdAddr/1
  Generate Output Control Signals/3(valid) -> valid/1
  Generate Output Control Signals/2(end) -> end/1
  Generate Output Control Signals/1(start) -> start/1
  Generate Read Address/2(currentAddr) -> Add1/1
  Generate Base Read Address/1(baseAddr) -> Delay1/1
  fifoData/1 -> Unit Delay Enabled Synchronous1/1
  Add1/1 -> Delay7/1
  Delay3/1 -> Relational Operator1/2
  MATLAB Function/1(out) -> Generate Read Address/2(enable), Delay2/1
  Unit Delay Enabled Synchronous1/1 -> Generate Read Address/1(blockLen), Delay4/1  "blockLen"
  Relational Operator1/1 -> Generate Read Address/3(reset), Generate Base Read Address/1(readStart), Unit Delay Enabled Synchronous1/2, MATLAB Function/1(trigger)  "readStart"
  fifoCount/1 -> Relational Operator1/1, Delay3/1

== system soc_WLAN_fpga/WLAN/WLAN HDL/WLAN_Tx_Rx/WLAN_Rx/WLANHDLReceiver/DataRecovery/Deinterleaver/DeInterleaver_HT/Stage 2 BPSK/Write Logic ==
  start : Inport
  valid : Inport  Port=2
  end : Inport  Port=3
  Generate Write Address : Subsystem
  Handle Input Control Signals : Subsystem
  wrAddr : Outport
  wrValid : Outport  Port=2
  count : Outport  Port=3
  endOut : Outport  Port=4
  endReady : Outport  Port=5
  wires:
  Handle Input Control Signals/4(endReady) -> endReady/1
  end/1 -> Handle Input Control Signals/3(end)
  valid/1 -> Handle Input Control Signals/2(valid)
  Generate Write Address/1(wrAddr) -> wrAddr/1
  Handle Input Control Signals/2(countEnb) -> Generate Write Address/2(enb), wrValid/1
  start/1 -> Handle Input Control Signals/1(start)
  Handle Input Control Signals/3(endOut) -> Generate Write Address/3(end), endOut/1
  Handle Input Control Signals/1(reset) -> Generate Write Address/1(rst)
  Generate Write Address/2(count) -> count/1

== system soc_WLAN_fpga/WLAN/WLAN HDL/WLAN_Tx_Rx/WLAN_Rx/WLANHDLReceiver/DataRecovery/Deinterleaver/DeInterleaver_HT/Stage 2 QPSK/Generate Ready ==
  advPop : Inport
  fifoCount : Inport  Port=2
  pop : Inport  Port=3
  endReady : Inport  Port=4
  Generate Ready2 : Subsystem
  Logical Operator1 : Logic  IconShape=distinctive  AllPortsSameDT=off  OutDataTypeStr=boolean
  Logical Operator2 : Logic  IconShape=distinctive  AllPortsSameDT=off  OutDataTypeStr=boolean
  Logical Operator3 : Logic  Operator=NOT  IconShape=distinctive  AllPortsSameDT=off  OutDataTypeStr=boolean
  MATLAB Function1 : MATLAB Function  TreatAsAtomicUnit=on  mask{nClocks=4}
      mask prompts: nClocks "Number of clocks to hold:"
  ready : Outport
  wires:
  pop/1 -> Generate Ready2/2(pop)
  Logical Operator3/1 -> Logical Operator2/2
  endReady/1 -> Logical Operator1/2
  MATLAB Function1/1(out) -> Logical Operator3/1
  fifoCount/1 -> Generate Ready2/1(fifoCount)
  Logical Operator1/1 -> MATLAB Function1/1(trigger)
  advPop/1 -> Logical Operator1/1
  Logical Operator2/1 -> ready/1
  Generate Ready2/1(ready2) -> Logical Operator2/1

== system soc_WLAN_fpga/WLAN/WLAN HDL/WLAN_Tx_Rx/WLAN_Rx/WLANHDLReceiver/DataRecovery/Deinterleaver/DeInterleaver_HT/Stage 2 QPSK/Read Logic ==
  fifoData : Inport
  fifoCount : Inport  Port=2
  Add1 : Sum  OutDataTypeStr=Inherit: Inherit via back propagation
  Delay1 : Delay  DelayLength=5
  Delay2 : Delay  DelayLength=5
  Delay3 : Delay  DelayLength=1
  Delay4 : Delay  DelayLength=5
  Delay7 : Delay  DelayLength=1
  Generate Base Read Address : Subsystem
  Generate Output Control Signals : Subsystem
  Generate Read Address : Subsystem  Variant=on
  MATLAB Function : MATLAB Function  TreatAsAtomicUnit=on  mask{nClocks=maxBlkSize}
      mask prompts: nClocks "Number of clocks to hold:"
  Relational Operator1 : RelationalOperator  Operator=<  OutDataTypeStr=boolean  InputSameDT=off
  Unit Delay Enabled Synchronous1 : hdlsllib/Discrete/Unit Delay Enabled Synchronous  InitialCondition=maxBlkSize -1  SampleTime=-1
  rdAddr : Outport
  start : Outport  Port=2
  end : Outport  Port=3
  valid : Outport  Port=4
  pop : Outport  Port=5
  advPop : Outport  Port=6
  wires:
  Generate Output Control Signals/5(advPop) -> advPop/1
  Generate Output Control Signals/4(pop) -> pop/1
  Delay1/1 -> Add1/2
  Generate Read Address/1(blockDataCount) -> Generate Output Control Signals/3(blockCount)
  Delay2/1 -> Generate Output Control Signals/2(blockValid)
  Delay4/1 -> Generate Output Control Signals/1(blockLen)
  Delay7/1 -> rdAddr/1
  Generate Output Control Signals/3(valid) -> valid/1
  Generate Output Control Signals/2(end) -> end/1
  Generate Output Control Signals/1(start) -> start/1
  Generate Read Address/2(currentAddr) -> Add1/1
  Generate Base Read Address/1(baseAddr) -> Delay1/1
  fifoData/1 -> Unit Delay Enabled Synchronous1/1
  Add1/1 -> Delay7/1
  Delay3/1 -> Relational Operator1/2
  MATLAB Function/1(out) -> Generate Read Address/2(enable), Delay2/1
  Unit Delay Enabled Synchronous1/1 -> Generate Read Address/1(blockLen), Delay4/1  "blockLen"
  Relational Operator1/1 -> Generate Read Address/3(reset), Generate Base Read Address/1(readStart), Unit Delay Enabled Synchronous1/2, MATLAB Function/1(trigger)  "readStart"
  fifoCount/1 -> Relational Operator1/1, Delay3/1

== system soc_WLAN_fpga/WLAN/WLAN HDL/WLAN_Tx_Rx/WLAN_Rx/WLANHDLReceiver/DataRecovery/Deinterleaver/DeInterleaver_HT/Stage 2 QPSK/Write Logic ==
  start : Inport
  valid : Inport  Port=2
  end : Inport  Port=3
  Generate Write Address : Subsystem
  Handle Input Control Signals : Subsystem
  wrAddr : Outport
  wrValid : Outport  Port=2
  count : Outport  Port=3
  endOut : Outport  Port=4
  endReady : Outport  Port=5
  wires:
  Handle Input Control Signals/4(endReady) -> endReady/1
  end/1 -> Handle Input Control Signals/3(end)
  valid/1 -> Handle Input Control Signals/2(valid)
  Generate Write Address/1(wrAddr) -> wrAddr/1
  Handle Input Control Signals/2(countEnb) -> Generate Write Address/2(enb), wrValid/1
  start/1 -> Handle Input Control Signals/1(start)
  Handle Input Control Signals/3(endOut) -> Generate Write Address/3(end), endOut/1
  Handle Input Control Signals/1(reset) -> Generate Write Address/1(rst)
  Generate Write Address/2(count) -> count/1

== system soc_WLAN_fpga/WLAN/WLAN HDL/WLAN_Tx_Rx/WLAN_Rx/WLANHDLReceiver/DataRecovery/Deinterleaver/DeInterleaver_NonHT/Stage 2 16QAM /Generate Ready ==
  advPop : Inport
  fifoCount : Inport  Port=2
  pop : Inport  Port=3
  endReady : Inport  Port=4
  Generate Ready2 : Subsystem
  Logical Operator1 : Logic  IconShape=distinctive  AllPortsSameDT=off  OutDataTypeStr=boolean
  Logical Operator2 : Logic  IconShape=distinctive  AllPortsSameDT=off  OutDataTypeStr=boolean
  Logical Operator3 : Logic  Operator=NOT  IconShape=distinctive  AllPortsSameDT=off  OutDataTypeStr=boolean
  MATLAB Function1 : MATLAB Function  TreatAsAtomicUnit=on  mask{nClocks=4}
      mask prompts: nClocks "Number of clocks to hold:"
  ready : Outport
  wires:
  pop/1 -> Generate Ready2/2(pop)
  Logical Operator3/1 -> Logical Operator2/2
  endReady/1 -> Logical Operator1/2
  MATLAB Function1/1(out) -> Logical Operator3/1
  fifoCount/1 -> Generate Ready2/1(fifoCount)
  Logical Operator1/1 -> MATLAB Function1/1(trigger)
  advPop/1 -> Logical Operator1/1
  Logical Operator2/1 -> ready/1
  Generate Ready2/1(ready2) -> Logical Operator2/1
